simulink model "quad_drag_ssmethod_tcurve"  (R2015b)
settings: Solver=VariableStepAuto  StartTime=0.0  StopTime=10  RelTol=1e-3
values from neighbouring files (symbols this model uses):
  breakpoints1 = data(end:-1:1,1)'    [Experimental_Impl.m]    (also in Experimental_Impl_wPlot.m; FEB02_LAKE_TEST.m; FEB14_LAKE_TEST.m; FEB28_LAKE_TEST.m)
  table_data = data(end:-1:1,2)'    [Experimental_Impl.m]    (also in Experimental_Impl_wPlot.m; FEB02_LAKE_TEST.m; FEB14_LAKE_TEST.m; FEB28_LAKE_TEST.m)
settings Model: Creator=bsb  LastModifiedBy=bsb
settings ConfigComp: CovModelRefEnable=Off
settings ConfigurationSet: Description=Simscape Multibody

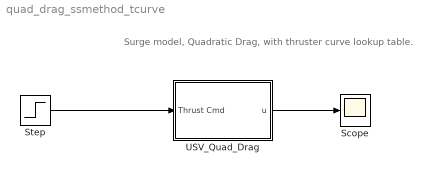
== system quad_drag_ssmethod_tcurve ==
  note: Surge model, Quadratic Drag, with thruster curve lookup table.
  Scope : Scope
  Step : Step  After=10  SampleTime=0
  USV_Quad_Drag : Subsystem
  wires:
  Step/1 -> USV_Quad_Drag/1(Thrust Cmd)
  USV_Quad_Drag/1(u) -> Scope/1

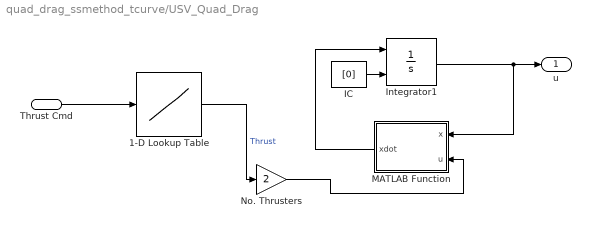
== system quad_drag_ssmethod_tcurve/USV_Quad_Drag ==
  Thrust Cmd : Inport
  1-D Lookup Table : Lookup_n-D  NumberOfTableDimensions=1  BreakpointsForDimension1=breakpoints1  Table=table_data  ExtrapMethod=Clip  UseLastTableValue=on  InternalRulePriority=Speed  RndMeth=Simplest  InputSameDT=on
  IC : Constant  Value=[0]
  Integrator1 : Integrator  InitialConditionSource=external
  MATLAB Function : MATLAB Function  TreatAsAtomicUnit=on
  No. Thrusters : Gain  Gain=2
  u : Outport
  wires:
  IC/1 -> Integrator1/2
  MATLAB Function/1(xdot) -> Integrator1/1
  Integrator1/1 -> u/1, MATLAB Function/1(x)
  No. Thrusters/1 -> MATLAB Function/2(u)
  1-D Lookup Table/1 -> No. Thrusters/1  "Thrust"
  Thrust Cmd/1 -> 1-D Lookup Table/1

== matlab function quad_drag_ssmethod_tcurve/USV_Quad_Drag/MATLAB Function ==
  data: x input; u input; xdot output
function xdot = fcn(x,u)
%#codegen

% x - state of the system.  surge velocity.
% u - input. thrust force
% Model parameters
m = 28.0;   % Mass [kg]
d = 16.9;  % Quadratic drag coefficient [N/(m/s)^2]

xdot = 1/m*(-d*abs(x)*x+u);
